simulink model "Q4_IIR_Direct_Realization"  (R2020b)
settings: Solver=VariableStepAuto  StartTime=0.0  StopTime=10.0  RelTol=1e-3
values from neighbouring files (symbols this model uses):
  a1 = 0.5    [data_dict.sldd]
  a2 = -0.25    [data_dict.sldd]
  b0 = 1.0    [data_dict.sldd]
  b1 = 0.4    [data_dict.sldd]
libraries: simulink x1
settings Model: DataDictionary=data_dict.sldd  Creator=Shree  LastModifiedBy=Shree

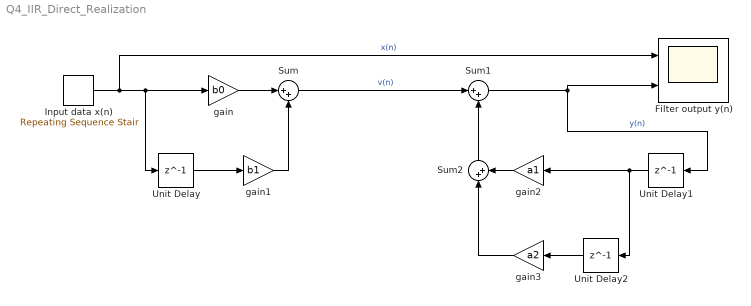
== system Q4_IIR_Direct_Realization ==
  Filter output y(n) : Scope  NumInputPorts=2
  Input data x(n) : simulink/Sources/Repeating Sequence Stair  OutValues=input  tsamp=-1  OutMin=[]  OutMax=[]  OutDataTypeStr=double  OutputDataTypeScalingMode=double  OutDataType=fixdt(0,8)  ConRadixGroup=Best Precision: Vector-wise  OutScaling=2^-12
  Sum : Sum  Inputs=|++
  Sum1 : Sum  Inputs=|++
  Sum2 : Sum  Inputs=|++
  Unit Delay : Delay  DelayLength=1  InitialCondition=0
  Unit Delay1 : Delay  DelayLength=1  InitialCondition=0
  Unit Delay2 : Delay  DelayLength=1  InitialCondition=0
  gain : Gain  Gain=b0
  gain1 : Gain  Gain=b1
  gain2 : Gain  Gain=a1
  gain3 : Gain  Gain=a2
  wires:
  Unit Delay/1 -> gain1/1
  Unit Delay1/1 -> Unit Delay2/1, gain2/1
  Unit Delay2/1 -> gain3/1
  gain1/1 -> Sum/2
  gain2/1 -> Sum2/2
  gain3/1 -> Sum2/1
  Sum2/1 -> Sum1/2
  Sum/1 -> Sum1/1  "v(n)"
  Input data x(n)/1 -> Filter output y(n)/1, Unit Delay/1, gain/1  "x(n)"
  Sum1/1 -> Unit Delay1/1, Filter output y(n)/2  "y(n)"
  gain/1 -> Sum/1
